simulink model "model"  (R2024a)
settings: Solver=VariableStepAuto  StartTime=0.0  StopTime=20  RelTol=1e-3
libraries: cstblocks x2
settings Model: SimulationMode=accelerator  Creator=thoma  LastModifiedBy=thoma

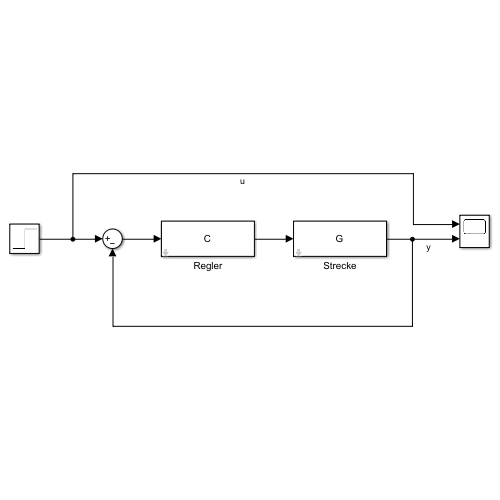
[thumbnail: Simulink's stored preview of the top-level diagram]
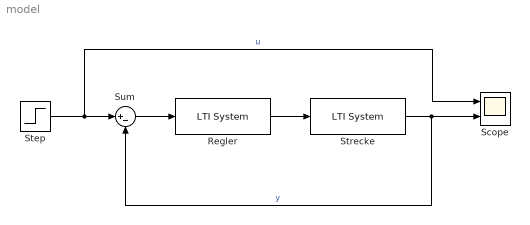
== system model ==
  Regler : cstblocks/LTI System  sys=C  IC=[]  PadeOrder=0
  Scope : Scope  NumInputPorts=2
  Step : Step  SampleTime=0
  Strecke : cstblocks/LTI System  sys=G  IC=[]  PadeOrder=0
  Sum : Sum  Inputs=|+-
  wires:
  Strecke/1 -> Sum/2, Scope/2  "y"
  Step/1 -> Sum/1, Scope/1  "u"
  Sum/1 -> Regler/1
  Regler/1 -> Strecke/1
